simulink model "BLDC_stern_state_space"  (R2018a)
settings: Solver=VariableStepAuto  StartTime=0.0  StopTime=10.0  RelTol=1e-3
values from neighbouring files (symbols this model uses):
  A = [-Rs/Ls,    0,      0,        0 ... (first row only)    [bldc_motor.m]    (also in test_simulink.m = 0.323; test_simulink_0.m = 2; ueb_simulink_ofen.m = 0.323)
  B = [2/(3*Ls), 1/(3*Ls),   0 ... (first row only)    [bldc_motor.m]
  C = [1, 0, 0, 0 ... (first row only)    [bldc_motor.m]    (also in test_simulink.m = 1)
  D = [0, 0, 0 ... (first row only)    [bldc_motor.m]
  M_Last = 0    [bldc_motor.m]
  p = 4    [bldc_motor.m]
  Psi_s = Psi/2    (= 0.01325)    [bldc_motor.m]
  U_B = 13    [bldc_motor.m]
settings Model: Creator=Dirk Horst  LastModifiedBy=Horst
settings CodeAppCC: StateflowObjectComments=on

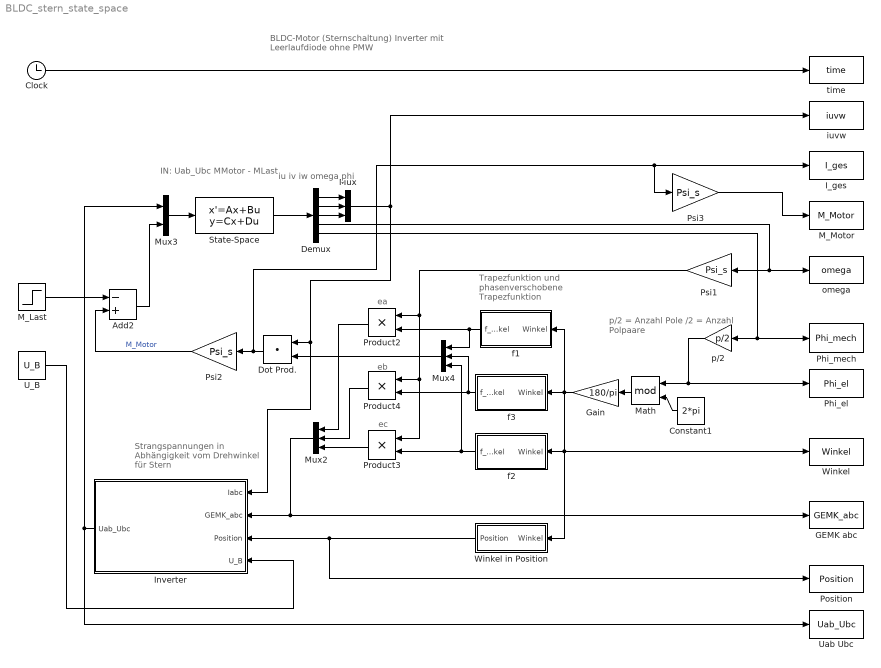
== system BLDC_stern_state_space ==
  note: BLDC-Motor (Sternschaltung)
      | Inverter mit Leerlaufdiode ohne PMW
  note: p/2 = Anzahl Pole /2
      | = Anzahl Polpaare
  note: ec
  note: eb
  note: ea
  note: IN: Uab_Ubc
      |      MMotor - MLast
  note: iu
      | iv
      | iw
      | omega
      | phi
  note: Strangspannungen
      | in Abhängigkeit vom
      | Drehwinkel für Stern
  note: Trapezfunktion und
      | phasenverschobene
      | Trapezfunktion
  Add2 : Sum  Inputs=-+
  Clock : Clock
  Constant1 : Constant  Value=2*pi
  Demux : Demux  Outputs=5
  Dot Prod. : DotProduct  InputSameDT=on  OutDataTypeStr=Inherit: Inherit via internal rule
  GEMK abc : ToWorkspace  VariableName=GEMK_abc  SampleTime=-1
      settings: Save2DSignal=2-D array (concatenate along first dimension)
  Gain : Gain  Gain=180/pi
  I_ges : ToWorkspace  VariableName=I_ges  SampleTime=-1
      settings: Save2DSignal=2-D array (concatenate along first dimension)
  Inverter : MATLAB Function  TreatAsAtomicUnit=on
  M_Last : Step  Time=0.001  After=M_Last  SampleTime=0
  M_Motor : ToWorkspace  VariableName=M_Motor  SampleTime=-1
      settings: Save2DSignal=2-D array (concatenate along first dimension)
  Math : Math  Operator=mod  SaturateOnIntegerOverflow=on
  Mux : Mux  Inputs=3
  Mux2 : Mux  Inputs=3
  Mux3 : Mux  Inputs=2
  Mux4 : Mux  Inputs=3
  Phi_el : ToWorkspace  VariableName=Phi_el  SampleTime=-1
      settings: Save2DSignal=2-D array (concatenate along first dimension)
  Phi_mech : ToWorkspace  VariableName=Phi_mech  SampleTime=-1
      settings: Save2DSignal=2-D array (concatenate along first dimension)
  Position : ToWorkspace  VariableName=Position  SampleTime=-1
      settings: Save2DSignal=2-D array (concatenate along first dimension)
  Product2 : Product
  Product3 : Product
  Product4 : Product
  Psi1 : Gain  Gain=Psi_s
  Psi2 : Gain  Gain=Psi_s
  Psi3 : Gain  Gain=Psi_s
  State-Space : StateSpace  A=A  B=B  C=C  D=D  InitialCondition=0
  U_B : Constant  Value=U_B
  Uab Ubc : ToWorkspace  VariableName=Uab_Ubc  SampleTime=-1
      settings: Save2DSignal=2-D array (concatenate along first dimension)
  Winkel : ToWorkspace  VariableName=Winkel  SampleTime=-1
  Winkel in Position : Subsystem
  f1 : Subsystem
  f2 : Subsystem
  f3 : Subsystem
  iuvw : ToWorkspace  VariableName=iuvw  SampleTime=-1
  omega : ToWorkspace  VariableName=omega  SampleTime=-1
  p/2 : Gain  Gain=p/2
  time : ToWorkspace  VariableName=time  SampleTime=-1
  wires:
  Mux/1 -> iuvw/1, Inverter/1(Iabc), Dot Prod./1
  Mux3/1 -> State-Space/1
  Demux/1 -> Mux/1
  Demux/2 -> Mux/2
  Demux/3 -> Mux/3
  Psi1/1 -> Product3/1, Product4/1, Product2/1
  Product2/1 -> Mux2/1
  Demux/4 -> omega/1, Psi1/1
  Constant1/1 -> Math/2
  Mux2/1 -> GEMK abc/1, Inverter/2(GEMK_abc)
  U_B/1 -> Inverter/4(U_B)
  Add2/1 -> Mux3/2
  f1/1(f_Winkel) -> Mux4/1, Product2/2
  f2/1(f_Winkel) -> Mux4/3, Product3/2
  f3/1(f_Winkel) -> Mux4/2, Product4/2
  Mux4/1 -> Dot Prod./2
  Winkel in Position/1(Position) -> Position/1, Inverter/3(Position)
  State-Space/1 -> Demux/1
  Demux/5 -> p/2/1, Phi_mech/1
  Product4/1 -> Mux2/2
  Product3/1 -> Mux2/3
  Dot Prod./1 -> Psi3/1, I_ges/1, Psi2/1
  Psi2/1 -> Add2/2  "M_Motor"
  p/2/1 -> Math/1, Phi_el/1
  M_Last/1 -> Add2/1
  Clock/1 -> time/1
  Gain/1 -> f3/1(Winkel), f1/1(Winkel), f2/1(Winkel), Winkel in Position/1(Winkel), Winkel/1
  Math/1 -> Gain/1
  Inverter/1(Uab_Ubc) -> Mux3/1, Uab Ubc/1
  Psi3/1 -> M_Motor/1

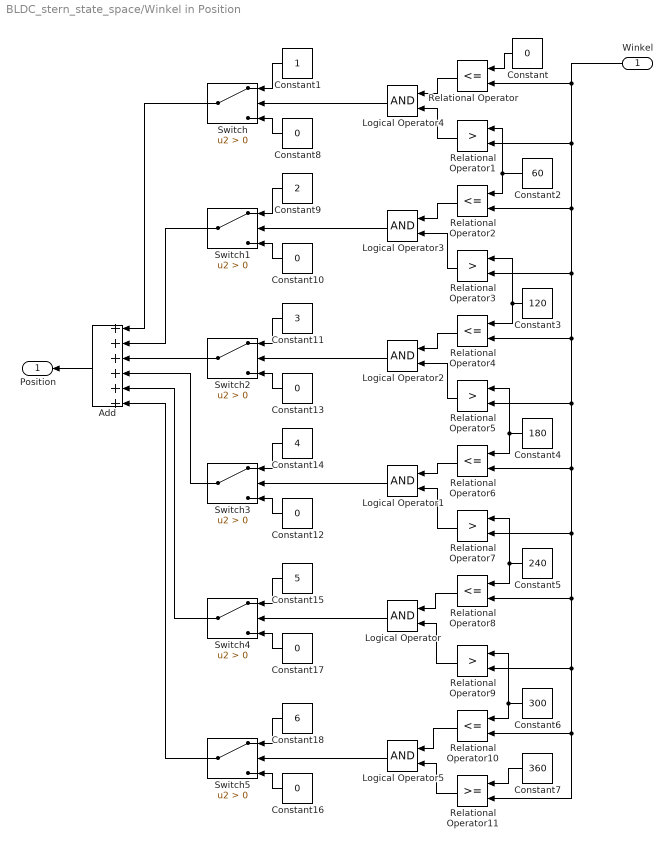
== system BLDC_stern_state_space/Winkel in Position ==
  Winkel : Inport
  Add : Sum  Inputs=++++++
  Constant{,8,10,12..13,16..17} (7 alike) : Constant  Value=0
  Constant1 : Constant
  Constant11 : Constant  Value=3
  Constant14 : Constant  Value=4
  Constant15 : Constant  Value=5
  Constant18 : Constant  Value=6
  Constant2 : Constant  Value=60
  Constant3 : Constant  Value=120
  Constant4 : Constant  Value=180
  Constant5 : Constant  Value=240
  Constant6 : Constant  Value=300
  Constant7 : Constant  Value=360
  Constant9 : Constant  Value=2
  Logical Operator{,1..5} (6 alike) : Logic  AllPortsSameDT=off  OutDataTypeStr=boolean
  Relational Operator{,2,4,6,8,10} (6 alike) : RelationalOperator  Operator=<=  OutDataTypeStr=boolean  RndMeth=Simplest
  Relational Operator{1,3,5,7,9} (5 alike) : RelationalOperator  Operator=>  OutDataTypeStr=boolean  RndMeth=Simplest
  Relational Operator11 : RelationalOperator  OutDataTypeStr=boolean  RndMeth=Simplest
  Switch{,1..5} (6 alike) : Switch  Criteria=u2 > Threshold
  Position : Outport
  wires:
  Constant5/1 -> Relational Operator8/1, Relational Operator7/1
  Constant4/1 -> Relational Operator5/1, Relational Operator6/1
  Relational Operator7/1 -> Logical Operator1/2
  Constant3/1 -> Relational Operator3/1, Relational Operator4/1
  Logical Operator4/1 -> Switch/2
  Relational Operator2/1 -> Logical Operator3/1
  Constant2/1 -> Relational Operator1/1, Relational Operator2/1
  Relational Operator3/1 -> Logical Operator3/2
  Relational Operator/1 -> Logical Operator4/1
  Constant6/1 -> Relational Operator9/1, Relational Operator10/1
  Relational Operator1/1 -> Logical Operator4/2
  Relational Operator8/1 -> Logical Operator/1
  Relational Operator4/1 -> Logical Operator2/1
  Relational Operator5/1 -> Logical Operator2/2
  Relational Operator6/1 -> Logical Operator1/1
  Relational Operator11/1 -> Logical Operator5/2
  Relational Operator10/1 -> Logical Operator5/1
  Relational Operator9/1 -> Logical Operator/2
  Constant7/1 -> Relational Operator11/1
  Winkel/1 -> Relational Operator/2, Relational Operator2/2, Relational Operator4/2, Relational Operator5/2, Relational Operator6/2, Relational Operator7/2, Relational Operator8/2, Relational Operator9/2, Relational Operator11/2, Relational Operator10/2, Relational Operator3/2, Relational Operator1/2
  Constant8/1 -> Switch/3
  Constant1/1 -> Switch/1
  Logical Operator3/1 -> Switch1/2
  Constant10/1 -> Switch1/3
  Constant9/1 -> Switch1/1
  Logical Operator2/1 -> Switch2/2
  Constant13/1 -> Switch2/3
  Constant11/1 -> Switch2/1
  Logical Operator1/1 -> Switch3/2
  Constant12/1 -> Switch3/3
  Constant14/1 -> Switch3/1
  Logical Operator/1 -> Switch4/2
  Constant17/1 -> Switch4/3
  Constant15/1 -> Switch4/1
  Logical Operator5/1 -> Switch5/2
  Constant16/1 -> Switch5/3
  Constant18/1 -> Switch5/1
  Add/1 -> Position/1
  Switch5/1 -> Add/6
  Switch4/1 -> Add/5
  Switch3/1 -> Add/4
  Switch2/1 -> Add/3
  Switch1/1 -> Add/2
  Switch/1 -> Add/1
  Constant/1 -> Relational Operator/1

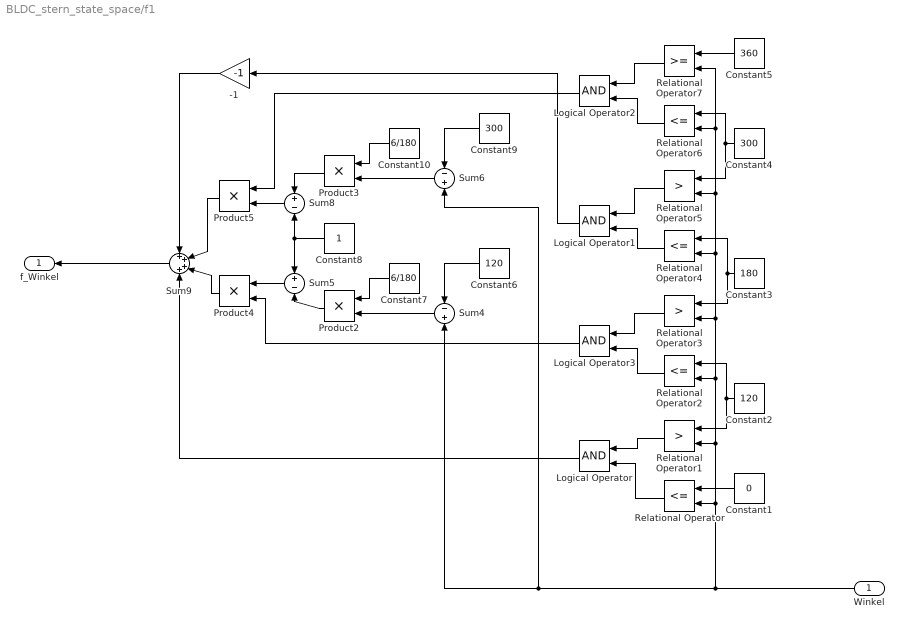
== system BLDC_stern_state_space/f1 ==
  Winkel : Inport
  -1 : Gain  Gain=-1
  Constant1 : Constant  Value=0
  Constant10 : Constant  Value=6/180
  Constant2 : Constant  Value=120
  Constant3 : Constant  Value=180
  Constant4 : Constant  Value=300
  Constant5 : Constant  Value=360
  Constant6 : Constant  Value=120
  Constant7 : Constant  Value=6/180
  Constant8 : Constant
  Constant9 : Constant  Value=300
  Logical Operator{,1..3} (4 alike) : Logic  AllPortsSameDT=off  OutDataTypeStr=boolean
  Product{2..5} (4 alike) : Product
  Relational Operator{,2,4,6} (4 alike) : RelationalOperator  Operator=<=  OutDataTypeStr=boolean  RndMeth=Simplest
  Relational Operator1 : RelationalOperator  Operator=>  OutDataTypeStr=boolean  RndMeth=Simplest
  Relational Operator3 : RelationalOperator  Operator=>  OutDataTypeStr=boolean  RndMeth=Simplest
  Relational Operator5 : RelationalOperator  Operator=>  OutDataTypeStr=boolean  RndMeth=Simplest
  Relational Operator7 : RelationalOperator  OutDataTypeStr=boolean  RndMeth=Simplest
  Sum4 : Sum  Inputs=-+
  Sum5 : Sum  Inputs=+-
  Sum6 : Sum  Inputs=-+
  Sum8 : Sum  Inputs=+-
  Sum9 : Sum  Inputs=++++
  f_Winkel : Outport
  wires:
  Constant5/1 -> Relational Operator7/1
  Constant7/1 -> Product2/1
  Relational Operator/1 -> Logical Operator/2
  Constant9/1 -> Sum6/1
  Product3/1 -> Sum8/1
  Sum6/1 -> Product3/2
  Constant10/1 -> Product3/1
  Relational Operator5/1 -> Logical Operator1/1
  Sum8/1 -> Product5/2
  Sum9/1 -> f_Winkel/1
  Logical Operator/1 -> Sum9/4
  Winkel/1 -> Relational Operator7/2, Relational Operator6/2, Relational Operator5/2, Relational Operator4/2, Relational Operator3/2, Relational Operator2/2, Relational Operator1/2, Relational Operator/2, Sum6/2, Sum4/2
  Sum4/1 -> Product2/2
  Relational Operator1/1 -> Logical Operator/1
  Constant6/1 -> Sum4/1
  Constant8/1 -> Sum8/2, Sum5/1
  Constant1/1 -> Relational Operator/1
  Logical Operator1/1 -> -1/1
  -1/1 -> Sum9/1
  Product5/1 -> Sum9/2
  Sum5/1 -> Product4/1
  Logical Operator2/1 -> Product5/1
  Constant2/1 -> Relational Operator2/1, Relational Operator1/1
  Product4/1 -> Sum9/3
  Product2/1 -> Sum5/2
  Relational Operator7/1 -> Logical Operator2/1
  Relational Operator3/1 -> Logical Operator3/1
  Relational Operator4/1 -> Logical Operator1/2
  Constant3/1 -> Relational Operator4/1, Relational Operator3/1
  Relational Operator2/1 -> Logical Operator3/2
  Relational Operator6/1 -> Logical Operator2/2
  Constant4/1 -> Relational Operator6/1, Relational Operator5/1
  Logical Operator3/1 -> Product4/2

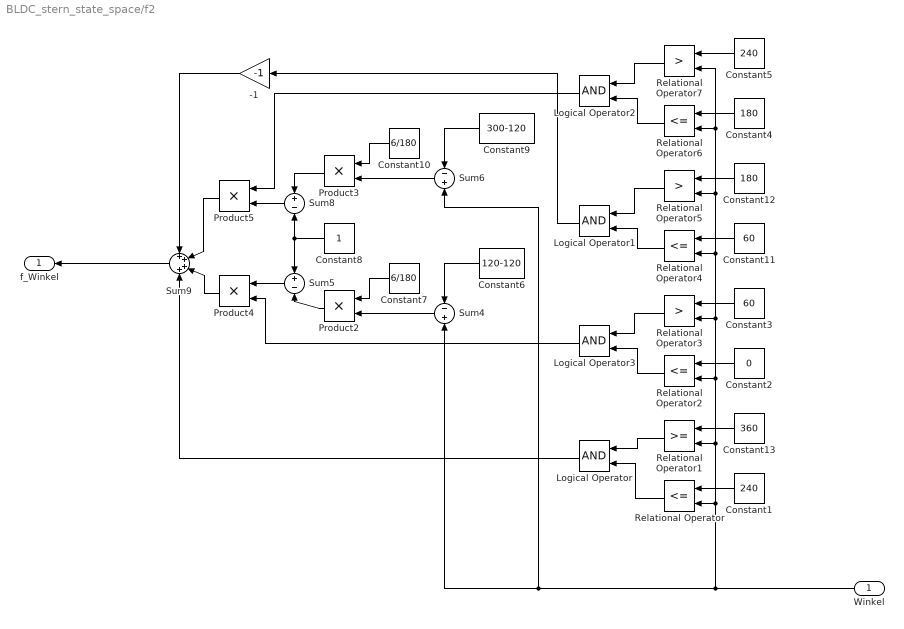
== system BLDC_stern_state_space/f2 ==
  Winkel : Inport
  -1 : Gain  Gain=-1
  Constant1 : Constant  Value=240
  Constant10 : Constant  Value=6/180
  Constant11 : Constant  Value=60
  Constant12 : Constant  Value=180
  Constant13 : Constant  Value=360
  Constant2 : Constant  Value=0
  Constant3 : Constant  Value=60
  Constant4 : Constant  Value=180
  Constant5 : Constant  Value=240
  Constant6 : Constant  Value=120-120
  Constant7 : Constant  Value=6/180
  Constant8 : Constant
  Constant9 : Constant  Value=300-120
  Logical Operator{,1..3} (4 alike) : Logic  AllPortsSameDT=off  OutDataTypeStr=boolean
  Product{2..5} (4 alike) : Product
  Relational Operator{,2,4,6} (4 alike) : RelationalOperator  Operator=<=  OutDataTypeStr=boolean  RndMeth=Simplest
  Relational Operator1 : RelationalOperator  OutDataTypeStr=boolean  RndMeth=Simplest
  Relational Operator3 : RelationalOperator  Operator=>  OutDataTypeStr=boolean  RndMeth=Simplest
  Relational Operator5 : RelationalOperator  Operator=>  OutDataTypeStr=boolean  RndMeth=Simplest
  Relational Operator7 : RelationalOperator  Operator=>  OutDataTypeStr=boolean  RndMeth=Simplest
  Sum4 : Sum  Inputs=-+
  Sum5 : Sum  Inputs=+-
  Sum6 : Sum  Inputs=-+
  Sum8 : Sum  Inputs=+-
  Sum9 : Sum  Inputs=++++
  f_Winkel : Outport
  wires:
  Product4/1 -> Sum9/3
  Product5/1 -> Sum9/2
  -1/1 -> Sum9/1
  Constant13/1 -> Relational Operator1/1
  Constant5/1 -> Relational Operator7/1
  Constant4/1 -> Relational Operator6/1
  Constant11/1 -> Relational Operator4/1
  Constant12/1 -> Relational Operator5/1
  Constant7/1 -> Product2/1
  Relational Operator/1 -> Logical Operator/2
  Constant9/1 -> Sum6/1
  Product3/1 -> Sum8/1
  Sum6/1 -> Product3/2
  Constant10/1 -> Product3/1
  Relational Operator5/1 -> Logical Operator1/1
  Sum8/1 -> Product5/2
  Sum9/1 -> f_Winkel/1
  Logical Operator/1 -> Sum9/4
  Winkel/1 -> Relational Operator7/2, Relational Operator6/2, Relational Operator5/2, Relational Operator4/2, Relational Operator3/2, Relational Operator2/2, Relational Operator1/2, Relational Operator/2, Sum6/2, Sum4/2
  Sum4/1 -> Product2/2
  Relational Operator1/1 -> Logical Operator/1
  Constant6/1 -> Sum4/1
  Constant8/1 -> Sum8/2, Sum5/1
  Constant1/1 -> Relational Operator/1
  Logical Operator1/1 -> -1/1
  Sum5/1 -> Product4/1
  Logical Operator2/1 -> Product5/1
  Constant2/1 -> Relational Operator2/1
  Product2/1 -> Sum5/2
  Relational Operator7/1 -> Logical Operator2/1
  Relational Operator3/1 -> Logical Operator3/1
  Relational Operator4/1 -> Logical Operator1/2
  Constant3/1 -> Relational Operator3/1
  Relational Operator2/1 -> Logical Operator3/2
  Relational Operator6/1 -> Logical Operator2/2
  Logical Operator3/1 -> Product4/2

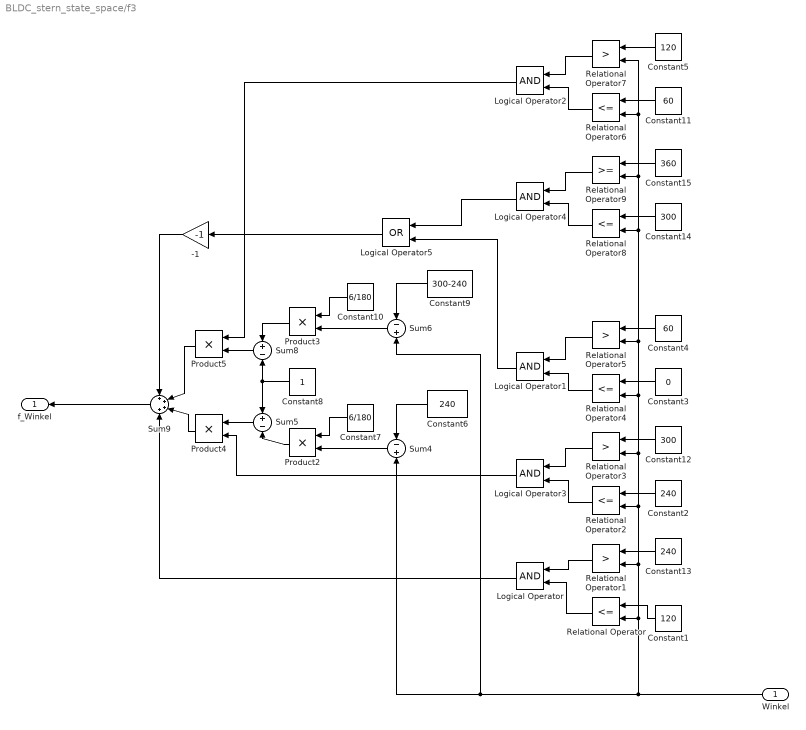
== system BLDC_stern_state_space/f3 ==
  Winkel : Inport
  -1 : Gain  Gain=-1
  Constant1 : Constant  Value=120
  Constant10 : Constant  Value=6/180
  Constant11 : Constant  Value=60
  Constant12 : Constant  Value=300
  Constant13 : Constant  Value=240
  Constant14 : Constant  Value=300
  Constant15 : Constant  Value=360
  Constant2 : Constant  Value=240
  Constant3 : Constant  Value=0
  Constant4 : Constant  Value=60
  Constant5 : Constant  Value=120
  Constant6 : Constant  Value=240
  Constant7 : Constant  Value=6/180
  Constant8 : Constant
  Constant9 : Constant  Value=300-240
  Logical Operator{,1..4} (5 alike) : Logic  AllPortsSameDT=off  OutDataTypeStr=boolean
  Logical Operator5 : Logic  Operator=OR  AllPortsSameDT=off  OutDataTypeStr=boolean
  Product{2..5} (4 alike) : Product
  Relational Operator{,2,4,6,8} (5 alike) : RelationalOperator  Operator=<=  OutDataTypeStr=boolean  RndMeth=Simplest
  Relational Operator{1,3,5,7} (4 alike) : RelationalOperator  Operator=>  OutDataTypeStr=boolean  RndMeth=Simplest
  Relational Operator9 : RelationalOperator  OutDataTypeStr=boolean  RndMeth=Simplest
  Sum4 : Sum  Inputs=-+
  Sum5 : Sum  Inputs=+-
  Sum6 : Sum  Inputs=-+
  Sum8 : Sum  Inputs=+-
  Sum9 : Sum  Inputs=++++
  f_Winkel : Outport
  wires:
  Logical Operator5/1 -> -1/1
  Logical Operator4/1 -> Logical Operator5/1
  Relational Operator9/1 -> Logical Operator4/1
  Relational Operator8/1 -> Logical Operator4/2
  Constant14/1 -> Relational Operator8/1
  Constant15/1 -> Relational Operator9/1
  Constant13/1 -> Relational Operator1/1
  Constant2/1 -> Relational Operator2/1
  Constant12/1 -> Relational Operator3/1
  Constant11/1 -> Relational Operator6/1
  Constant3/1 -> Relational Operator4/1
  Constant5/1 -> Relational Operator7/1
  Constant7/1 -> Product2/1
  Relational Operator/1 -> Logical Operator/2
  Constant9/1 -> Sum6/1
  Product3/1 -> Sum8/1
  Sum6/1 -> Product3/2
  Constant10/1 -> Product3/1
  Relational Operator5/1 -> Logical Operator1/1
  Sum8/1 -> Product5/2
  Sum9/1 -> f_Winkel/1
  Logical Operator/1 -> Sum9/4
  Winkel/1 -> Relational Operator5/2, Relational Operator8/2, Relational Operator9/2, Relational Operator7/2, Relational Operator6/2, Relational Operator4/2, Relational Operator3/2, Relational Operator2/2, Relational Operator1/2, Relational Operator/2, Sum6/2, Sum4/2
  Sum4/1 -> Product2/2
  Relational Operator1/1 -> Logical Operator/1
  Constant6/1 -> Sum4/1
  Constant8/1 -> Sum8/2, Sum5/1
  Constant1/1 -> Relational Operator/1
  Logical Operator1/1 -> Logical Operator5/2
  -1/1 -> Sum9/1
  Product5/1 -> Sum9/2
  Sum5/1 -> Product4/1
  Logical Operator2/1 -> Product5/1
  Product4/1 -> Sum9/3
  Product2/1 -> Sum5/2
  Relational Operator7/1 -> Logical Operator2/1
  Relational Operator3/1 -> Logical Operator3/1
  Relational Operator4/1 -> Logical Operator1/2
  Relational Operator2/1 -> Logical Operator3/2
  Relational Operator6/1 -> Logical Operator2/2
  Constant4/1 -> Relational Operator5/1
  Logical Operator3/1 -> Product4/2

== matlab function BLDC_stern_state_space/Inverter ==
  data: Iabc input; GEMK_abc input; Position input; Uab_Ubc output; U_B input
function Uab_Ubc = InverterStern01(Iabc,GEMK_abc, Position, U_B )

% Abhängig von der Rotorspannung werden die Summenspannungen für das
% Zustandsraum-Modell berechnet.
% Die Fallunterscheidung für die Position 2, 4 und 6 wurden gegenüber der
% Tabelle Seite 23 vertauscht. Warum das so sein muss weiß ich noch nicht.
%	
% Autor:	Horst Rumpf

%           
% Datum:    2017-10-16
%
% Änderung: 
%
% siehe auch: 02_BLDC_motor_Vorueberlegungen.pptx 
%--------------------------------------------------------------------------

% Initialisation (muss! sonst gibt es eine Fehlermeldung oder 
%                       unter otherwise Werte zuordnen)
Uab=0;
Ubc=0;  

ea=GEMK_abc(1); % EMK Strang a
eb=GEMK_abc(2); % EMK Strang b
ec=GEMK_abc(3); % EMK Strang c

%Phasenströme
Ia=Iabc(1);
Ib=Iabc(2);
Ic=Iabc(3);

%Mit oder ohne Freilaufdioden
Diod_yn=1;

if Diod_yn==1
if Ia <= 0
    IaZero=1;
else
    IaZero=0;
end

if Ib <=0
    IbZero=1;
else
    IbZero=0;
end


if Ic <=0
    IcZero=1;
else
    IcZero=0;
end

else
IaZero=1;
IbZero=1;
IcZero=1;
end


switch(Position)
    case 1  % 0° bis 60°
    %===================    
        if IcZero==1 % Ic == 0
            Uab=      U_B-ea+eb;
            Ubc=1/2*(-U_B+ea-eb);
        else
             Uab=      U_B-ea+eb;
            Ubc=          -eb+ec;
        end    
    case 2  % 60° bis 120°
    %=====================    
        if IbZero==1 % Ib == 0
            Uab=   -ea+eb;
            Ubc=U_B-eb+ec;
        else
            Uab=1/2*(U_B-ea+ec);
            Ubc=1/2*(U_B-ea+ec);  
        end    
            
    case 3  % 120° bis 180°
    %======================    
        if IaZero==1 % Ia == 0
            Uab=1/2*(-U_B+eb-ec);
            Ubc=      U_B-eb+ec;
        else
             Uab=-U_B-ea+eb;
             Ubc= U_B-eb+ec;
        end    
    case 4  % 180° bis 240°
    %======================    
        if IcZero==1 % Ic == 0
            Uab=-U_B-ea+eb;
            Ubc=     -eb+ec;
        else
            Uab=    -U_B-ea+eb;
            Ubc=1/2*(U_B+ea-eb);
        end    
    case 5  % 240° bis 300°
    %======================    
        if IbZero==1 % Ib == 0
            Uab=1/2*(-U_B-ea+ec);
            Ubc=1/2*(-U_B-ea+ec);
        else
             Uab=   -ea+eb;
            Ubc=-U_B-eb+ec;
        end    
    case 6  % 300° bis 360°
    %======================    
        if IaZero==1 % Ia == 0
             Uab= U_B-ea+eb;
            Ubc=-U_B-eb+ec;
        else
            Uab=1/2*(U_B+eb-ec);
            Ubc=    -U_B-eb+ec; 
        end        
     otherwise % Fehler, wenn Postion auf 0
     %========    
         disp('Position nicht 1 bis 6');
end     


    Uab_Ubc=[Uab, Ubc]';
